simulink model "rameno_2D"  (R2023a)
settings: Solver=VariableStepAuto  StartTime=0.0  StopTime=1.5  MaxStep=0.001  RelTol=1e-3  AbsTol=1e-3  EnableMultiTasking=on
InitFcn:
  | parameters;
values from neighbouring files (symbols this model uses):
  akt = u'    [optim_control_nlmpc.m]    (also in parameters.m = rand(1,15)*0)
  Ic = in3(:,4)    [MM.m]    (also in optim_control_nlmpc.m = 0.1; parameters.m = 0.01)
  Ih = in3(:,6)    [MM.m]    (also in optim_control_nlmpc.m = 0.3; parameters.m = 0.03)
  Is = in3(:,5)    [MM.m]    (also in optim_control_nlmpc.m = 0.2; parameters.m = 0.02)
  mc = in3(:,1)    [FO.m]    (also in MM.m; optim_control_nlmpc.m = 1; parameters.m = 0.074001)
  mh = in3(:,3)    [FO.m]    (also in MM.m; optim_control_nlmpc.m = 3; parameters.m = 2)
  ms = in3(:,2)    [FO.m]    (also in MM.m; optim_control_nlmpc.m = 2; parameters.m = 0.25518)
  x0 = [-0.0267856484256359	-0.0830006989527777	0.0354624220509602 0 0 0]'    [parameters.m]
undefined symbols (not defined in the file or in its folder): data, muscles, X, Y, Z
libraries: sm_lib x109, nesl_utility x33
(part 3 of 3)

== system rameno_2D/Muscles/Trapezius4 ==
  Aktivace : Inport
  Active_factor_norm : MATLAB Function  TreatAsAtomicUnit=on
  F0M : Gain  Gain=muscles.F0M(7)
  Graphic : sm_lib/Body Elements/Graphic  GraphicType=Marker  MarkerShape=Sphere  MarkerSize=10  GraphicVisPropType=SimpleVisualProperties  GraphicDiffuseColor=[0 1 1]  GraphicSpecularColor=[0.5 0.5 0.5 1.0]  GraphicAmbientColor=[0.15 0.15 0.15 1.0]  GraphicEmissiveColor=[0.0 0.0 0.0 1.0]  GraphicShininess=75  GraphicOpacity=1.0
  Graphic1 : sm_lib/Body Elements/Graphic  GraphicType=Marker  MarkerShape=Sphere  MarkerSize=10  GraphicVisPropType=SimpleVisualProperties  GraphicDiffuseColor=[0.05882 1 1]  GraphicSpecularColor=[0.5 0.5 0.5 1.0]  GraphicAmbientColor=[0.15 0.15 0.15 1.0]  GraphicEmissiveColor=[0.0 0.0 0.0 1.0]  GraphicShininess=75  GraphicOpacity=1.0
  Internal Force : sm_lib/Forces and Torques/Internal Force
  PECM1_1 : sm_lib/Frames and Transforms/Rigid Transform  TranslationMethod=Cartesian  TranslationStandardOffset=0  TranslationStandardOffsetUnits=m  TranslationStandardAxis=+Z  TranslationCartesianOffset=[muscles.origin(7,:)]  TranslationCartesianOffsetUnits=m  TranslationROffset=0  TranslationROffsetUnits=m  TranslationZOffset=0  TranslationZOffsetUnits=m  TranslationThetaOffset=0  TranslationThetaOffsetUnits=deg  RotationMethod=None  RotationAngleUnits=deg  RotationStandardAxis=+Z  RotationAngle=0.0  RotationArbitraryAxis=[0 0 1]  FollAlignAxisA=+X  BaseAlignAxisA=+Y  FollAlignAxisB=+Y  BaseAlignAxisB=+Z  RotationSequenceAxes=FollowerAxes  RotationSequence=XYX  RotationSequenceAngles=[0 0 0]  RotationSequenceAnglesUnits=deg  RotationMatrix=[1 0 0; 0 1 0; 0 0 1]  Quaternion=[1 0 0 0]
  PECM1_2 : sm_lib/Frames and Transforms/Rigid Transform  TranslationMethod=Cartesian  TranslationStandardOffset=0  TranslationStandardOffsetUnits=m  TranslationStandardAxis=+Z  TranslationCartesianOffset=[muscles.insertion(7,:)]  TranslationCartesianOffsetUnits=m  TranslationROffset=0  TranslationROffsetUnits=m  TranslationZOffset=0  TranslationZOffsetUnits=m  TranslationThetaOffset=0  TranslationThetaOffsetUnits=deg  RotationMethod=None  RotationAngleUnits=deg  RotationStandardAxis=+Y  RotationAngle=90  RotationArbitraryAxis=[0 0 1]  FollAlignAxisA=+X  BaseAlignAxisA=+Y  FollAlignAxisB=+Y  BaseAlignAxisB=+Z  RotationSequenceAxes=FollowerAxes  RotationSequence=XYX  RotationSequenceAngles=[0 0 0]  RotationSequenceAnglesUnits=deg  RotationMatrix=[1 0 0; 0 1 0; 0 0 1]  Quaternion=[1 0 0 0]
  PS-Simulink Converter : nesl_utility/PS-Simulink Converter  PhysicalDomain=network_engine_domain  SubClassName=ps_output  LeftPortType=input  RightPortType=output  PseudoPeriodic=off  Frequencies=[]  VectorFormat=inherit  Unit=inherit  AffineConversion=off
  Passive_force_norm : MATLAB Function  TreatAsAtomicUnit=on
  Scope : Scope
  Simulink-PS Converter : nesl_utility/Simulink-PS Converter  PhysicalDomain=network_engine_domain  SubClassName=ps_input  LeftPortType=input  RightPortType=output  PseudoPeriodic=off  Frequencies=[]  NoiseDistribution=none  NoiseParameters=[]  Unit=1  AffineConversion=off  FilteringAndDerivatives=provide  SimscapeFilterOrder=1  InputFilterTimeConstant=0.001  UdotUserProvided=0
  Sum : Sum  Inputs=|++
  Tlak->Tah : Gain
  Transform Sensor : sm_lib/Frames and Transforms/Transform Sensor  MeasurementFrame=World  RotationSequence=XYX  SenseAngle=off  SenseAxis=off  SenseQ=off  SenseR=off  SenseRotationSequence=off  SenseOmegaX=off  SenseOmegaY=off  SenseOmegaZ=off  SenseQDot=off  SenseRDot=off  SenseRotationSequenceDot=off  SenseAlphaX=off  SenseAlphaY=off  SenseAlphaZ=off  SenseQDDot=off  SenseRDDot=off  SenseX=off  SenseY=off  SenseZ=off  SenseRad=off  SenseAzim=off  SenseDist=on  SenseInc=off  SenseXDot=off  SenseYDot=off  SenseZDot=off  SenseRadDot=off  SenseAzimDot=off  SenseDistDot=off  SenseIncDot=off  SenseXDDot=off  SenseYDDot=off  SenseZDDot=off  SenseRadDDot=off  SenseAzimDDot=off  SenseDistDDot=off  SenseIncDDot=off
  force : Scope
  l0m : Constant  Value=muscles.L0M(7)
  Thorax : PMIOPort  Side=Left
  scapula : PMIOPort  Port=2  Side=Left
  wires:
  Sum/1 -> F0M/1
  F0M/1 -> Tlak->Tah/1
  Passive_force_norm/1(Fp_norm) -> Sum/1
  Active_factor_norm/1(Fa_norm) -> Sum/2
  Tlak->Tah/1 -> Simulink-PS Converter/1, force/1
  PS-Simulink Converter/1 -> Scope/1, Active_factor_norm/1(lm), Passive_force_norm/1(lm)
  l0m/1 -> Active_factor_norm/2(l0), Passive_force_norm/2(l0)
  Aktivace/1 -> Active_factor_norm/3(a)
  connections:
  Internal Force/LConn1 -- Transform Sensor/LConn1 -- Graphic1/RConn1 -- PECM1_2/RConn1
  Internal Force/RConn1 -- PECM1_1/RConn1 -- Graphic/RConn1 -- Transform Sensor/RConn1
  Simulink-PS Converter/RConn1 -- Internal Force/LConn2
  Transform Sensor/RConn2 -- PS-Simulink Converter/LConn1
  PECM1_1/LConn1 -- Thorax/RConn1
  PECM1_2/LConn1 -- scapula/RConn1

== matlab function rameno_2D/Muscles/PECM1/Active_factor_norm ==
  data: Fa_norm output; lm input; l0 input; a input
function Fa_norm = fcn(lm,l0,a)
f_gauss = 0.25;
Fa_norm = (exp(-(lm/l0-1)^2/f_gauss))*a;

== matlab function rameno_2D/Muscles/DELT/Active_factor_norm ==
  data: Fa_norm output; lm input; l0 input; a input
function Fa_norm = fcn(lm,l0,a)
f_gauss = 0.25;
Fa_norm = (exp(-(lm/l0-1)^2/f_gauss))*a;

== matlab function rameno_2D/Muscles/DELT/Passive_force_norm ==
  data: lm input; Fp_norm output; l0 input
function Fp_norm = fcn(lm,l0)
Fp_norm = ((lm/l0)^3)*exp(8*lm/l0-12.9);

== matlab function rameno_2D/Muscles/DELT/MATLAB Function ==
  data: u input; length output; muscles parameter; data parameter
function length = muscle_length(u,muscles, data)
length = 0;
length = muscle_length(3,4,muscles.origin(2,:),muscles.insertion(2,:),[0,0,u],1,data);

end

== matlab function rameno_2D/Muscles/Supraspinatus/Active_factor_norm ==
  data: Fa_norm output; lm input; l0 input; a input
function Fa_norm = fcn(lm,l0,a)
f_gauss = 0.25;
Fa_norm = (exp(-(lm/l0-1)^2/f_gauss))*a;

== matlab function rameno_2D/Muscles/Supraspinatus/Passive_force_norm ==
  data: lm input; Fp_norm output; l0 input
function Fp_norm = fcn(lm,l0)
Fp_norm = ((lm/l0)^3)*exp(8*lm/l0-12.9);

== matlab function rameno_2D/Muscles/Trapezius4/Active_factor_norm ==
  data: Fa_norm output; lm input; l0 input; a input
function Fa_norm = fcn(lm,l0,a)
f_gauss = 0.25;
Fa_norm = (exp(-(lm/l0-1)^2/f_gauss))*a;

== matlab function rameno_2D/Muscles/Trapezius4/Passive_force_norm ==
  data: lm input; Fp_norm output; l0 input
function Fp_norm = fcn(lm,l0)
Fp_norm = ((lm/l0)^3)*exp(8*lm/l0-12.9);

== matlab function rameno_2D/Muscles/Rhomboideus/Active_factor_norm ==
  data: Fa_norm output; lm input; l0 input; a input
function Fa_norm = fcn(lm,l0,a)
f_gauss = 0.25;
Fa_norm = (exp(-(lm/l0-1)^2/f_gauss))*a;

== matlab function rameno_2D/Muscles/Rhomboideus/Passive_force_norm ==
  data: lm input; Fp_norm output; l0 input
function Fp_norm = fcn(lm,l0)
Fp_norm = ((lm/l0)^3)*exp(8*lm/l0-12.9);

== matlab function rameno_2D/Muscles/PECM1/Passive_force_norm ==
  data: lm input; Fp_norm output; l0 input
function Fp_norm = fcn(lm,l0)
Fp_norm = ((lm/l0)^3)*exp(8*lm/l0-12.9);

== matlab function rameno_2D/Sympy EOMs ==
  data: t input; dy output; y input; data parameter; muscles parameter; akt input
% function dy = fcn(t,y,koef,SC_AC,c_COM, AC_GH, s_COM, h_COM)
function dy = fcn(t,y,data,muscles,akt)
dy = zeros(6,1);
SC_AC = data.SC_AC;
c_COM = data.c_COM;
AC_GH = data.AC_GH;
s_COM = data.s_COM;
h_COM = data.h_COM;
koef = data.koef;
mm = MM(t,y,koef,SC_AC,c_COM,AC_GH,s_COM,h_COM);
fo = FO(t,y,koef,SC_AC,c_COM,AC_GH,s_COM,h_COM);
fe = FE(t,y,muscles.F0M',muscles.L0M',akt');
dy = real(mm\(fo+fe));

== matlab function rameno_2D/Muscles/Trapezius1/Active_factor_norm ==
  data: Fa_norm output; lm input; l0 input; a input
function Fa_norm = fcn(lm,l0,a)
f_gauss = 0.25;
Fa_norm = (exp(-(lm/l0-1)^2/f_gauss))*a;

== matlab function rameno_2D/Muscles/PECM2/Active_factor_norm ==
  data: Fa_norm output; lm input; l0 input; a input
function Fa_norm = fcn(lm,l0,a)
f_gauss = 0.25;
Fa_norm = (exp(-(lm/l0-1)^2/f_gauss))*a;

== matlab function rameno_2D/Muscles/PECM2/Passive_force_norm ==
  data: lm input; Fp_norm output; l0 input
function Fp_norm = fcn(lm,l0)
Fp_norm = ((lm/l0)^3)*exp(8*lm/l0-12.9);

== matlab function rameno_2D/Muscles/PECM3/Active_factor_norm ==
  data: Fa_norm output; lm input; l0 input; a input
function Fa_norm = fcn(lm,l0,a)
f_gauss = 0.25;
Fa_norm = (exp(-(lm/l0-1)^2/f_gauss))*a;

== matlab function rameno_2D/Muscles/PECM3/Passive_force_norm ==
  data: lm input; Fp_norm output; l0 input
function Fp_norm = fcn(lm,l0)
Fp_norm = ((lm/l0)^3)*exp(8*lm/l0-12.9);

== matlab function rameno_2D/Muscles/Serr1/Active_factor_norm ==
  data: Fa_norm output; lm input; l0 input; a input
function Fa_norm = fcn(lm,l0,a)
f_gauss = 0.25;
Fa_norm = (exp(-(lm/l0-1)^2/f_gauss))*a;

== matlab function rameno_2D/Muscles/Serr1/Passive_force_norm ==
  data: lm input; Fp_norm output; l0 input
function Fp_norm = fcn(lm,l0)
Fp_norm = ((lm/l0)^3)*exp(8*lm/l0-12.9);

== matlab function rameno_2D/Muscles/Serr2/Active_factor_norm ==
  data: Fa_norm output; lm input; l0 input; a input
function Fa_norm = fcn(lm,l0,a)
f_gauss = 0.25;
Fa_norm = (exp(-(lm/l0-1)^2/f_gauss))*a;

== matlab function rameno_2D/Muscles/Serr2/Passive_force_norm ==
  data: lm input; Fp_norm output; l0 input
function Fp_norm = fcn(lm,l0)
Fp_norm = ((lm/l0)^3)*exp(8*lm/l0-12.9);

== matlab function rameno_2D/Muscles/Serr3/Active_factor_norm ==
  data: Fa_norm output; lm input; l0 input; a input
function Fa_norm = fcn(lm,l0,a)
f_gauss = 0.25;
Fa_norm = (exp(-(lm/l0-1)^2/f_gauss))*a;

== matlab function rameno_2D/Muscles/Serr3/Passive_force_norm ==
  data: lm input; Fp_norm output; l0 input
function Fp_norm = fcn(lm,l0)
Fp_norm = ((lm/l0)^3)*exp(8*lm/l0-12.9);

== matlab function rameno_2D/Muscles/Trapezius1/Passive_force_norm ==
  data: lm input; Fp_norm output; l0 input
function Fp_norm = fcn(lm,l0)
Fp_norm = ((lm/l0)^3)*exp(8*lm/l0-12.9);

== matlab function rameno_2D/Muscles/Levator/Active_factor_norm ==
  data: Fa_norm output; lm input; l0 input; a input
function Fa_norm = fcn(lm,l0,a)
f_gauss = 0.25;
Fa_norm = (exp(-(lm/l0-1)^2/f_gauss))*a;

== matlab function rameno_2D/Muscles/Levator/Passive_force_norm ==
  data: lm input; Fp_norm output; l0 input
function Fp_norm = fcn(lm,l0)
Fp_norm = ((lm/l0)^3)*exp(8*lm/l0-12.9);

== matlab function rameno_2D/Muscles/TerMin/Active_factor_norm ==
  data: Fa_norm output; lm input; l0 input; a input
function Fa_norm = fcn(lm,l0,a)
f_gauss = 0.25;
Fa_norm = (exp(-(lm/l0-1)^2/f_gauss))*a;

== matlab function rameno_2D/Muscles/TerMin/Passive_force_norm ==
  data: lm input; Fp_norm output; l0 input
function Fp_norm = fcn(lm,l0)
Fp_norm = ((lm/l0)^3)*exp(8*lm/l0-12.9);

== matlab function rameno_2D/Muscles/Trapezius2/Active_factor_norm ==
  data: Fa_norm output; lm input; l0 input; a input
function Fa_norm = fcn(lm,l0,a)
f_gauss = 0.25;
Fa_norm = (exp(-(lm/l0-1)^2/f_gauss))*a;

== matlab function rameno_2D/Muscles/Trapezius2/Passive_force_norm ==
  data: lm input; Fp_norm output; l0 input
function Fp_norm = fcn(lm,l0)
Fp_norm = ((lm/l0)^3)*exp(8*lm/l0-12.9);

== matlab function rameno_2D/Muscles/Trapezius3/Active_factor_norm ==
  data: Fa_norm output; lm input; l0 input; a input
function Fa_norm = fcn(lm,l0,a)
f_gauss = 0.25;
Fa_norm = (exp(-(lm/l0-1)^2/f_gauss))*a;

== matlab function rameno_2D/Muscles/Trapezius3/Passive_force_norm ==
  data: lm input; Fp_norm output; l0 input
function Fp_norm = fcn(lm,l0)
Fp_norm = ((lm/l0)^3)*exp(8*lm/l0-12.9);
